simulink model "Controller29_05"  (R2019b)
settings: Solver=VariableStepAuto  StartTime=0.0  StopTime=10.0  RelTol=1e-3
undefined symbols (not defined in the file): maxsteer, x_p, y_p
settings Model: Creator=s161230  LastModifiedBy=s161230

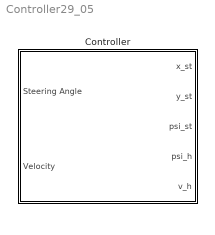
== system Controller29_05 ==
  Controller : Subsystem

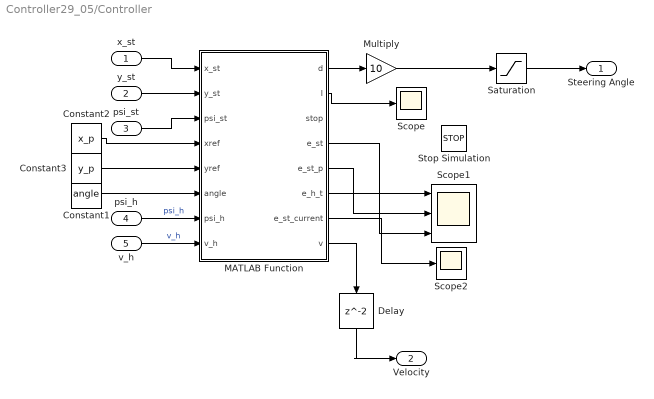
== system Controller29_05/Controller ==
  x_st : Inport  OutDataTypeStr=double
  y_st : Inport  Port=2  OutDataTypeStr=double
  psi_st : Inport  Port=3  OutDataTypeStr=double
  psi_h : Inport  Port=4  OutDataTypeStr=double
  v_h : Inport  Port=5  OutDataTypeStr=double
  Constant1 : Constant  Value=angle
  Constant2 : Constant  Value=x_p
  Constant3 : Constant  Value=y_p
  Delay : Delay  InitialCondition=-1.0
  MATLAB Function : MATLAB Function  TreatAsAtomicUnit=on
  Multiply : Gain  Gain=10
  Saturation : Saturate  UpperLimit=maxsteer  LowerLimit=-maxsteer  ZeroCross=off
  Scope : Scope
  Scope1 : Scope  NumInputPorts=3
  Scope2 : Scope
  Stop Simulation : Stop
  Steering Angle : Outport  OutDataTypeStr=double
  "Velocity " : Outport  Port=2
  wires:
  Constant1/1 -> MATLAB Function/6(angle)
  MATLAB Function/1(d) -> Multiply/1
  Constant2/1 -> MATLAB Function/4(xref)
  psi_st/1 -> MATLAB Function/3(psi_st)
  Constant3/1 -> MATLAB Function/5(yref)
  x_st/1 -> MATLAB Function/1(x_st)
  y_st/1 -> MATLAB Function/2(y_st)
  psi_h/1 -> MATLAB Function/7(psi_h)  "psi_h"
  v_h/1 -> MATLAB Function/8(v_h)  "v_h"
  Multiply/1 -> Saturation/1
  MATLAB Function/2(I) -> Scope/1
  MATLAB Function/4(e_st) -> Scope1/1
  MATLAB Function/5(e_st_p) -> Scope1/2
  MATLAB Function/6(e_h_t) -> Scope1/3
  Saturation/1 -> Steering Angle/1
  MATLAB Function/7(e_st_current) -> Scope2/1
  MATLAB Function/8(v) -> Delay/1
  Delay/1 -> "Velocity "/1

== matlab function Controller29_05/Controller/MATLAB Function ==
  data: d output; I output; stop output; x_st input; y_st input; psi_st input; xref input; yref input; angle input; psi_h input; v_h input; e_st output; e_st_p output; e_h_t output; e_st_current output; v output
function [d, I, stop, e_st, e_st_p, e_h_t, e_st_current, v]  = Error(x_st, y_st, psi_st, xref, yref, angle, psi_h,v_h)
    [~, I] = min(sqrt((xref-x_st).^2+(yref-y_st).^2));
    lookahead = 200;
    K1 = 80;%2
    K2 = 7.6;%13
    l_h = 0.22;
    l_st = 0.72;
    
    %1.0m
    lookahead = 77; %77
    K1 = 75;        %75
    K2 = 12;        %12
    
    %0.9m
    lookahead = 82;
    K1 = 76;
    K2 = 12;
    
    %0.8m
    lookahead = 86;
    K1 = 77;
    K2 = 12;
        
    %0.7m
    lookahead = 88;
    K1 = 79;
    K2 = 12;
    
    %0.6m
    lookahead = 95;
    K1 = 79;
    K2 = 12;
    
    %0.5m
    lookahead = 110;
    K1 = 79;
    K2 = 12;
    
    %0.4m
    lookahead = 150;
    K1 = 79;
    K2 = 12;
    
    %0.35m
%     lookahead = 210;
%     K1 = 86;
%     K2 = 12;
    
    %0.3m
%     lookahead = 220;
%     K1 = 90;
%     K2 = 12;
%     
    if I < length(angle) - 1
        stop = 0;
        
        if I < length(angle) - lookahead
            
             e_st_current = -sin(psi_st)*(x_st-xref(I))+cos(psi_st)*(y_st-yref(I));
             %define errors
             e_st = -sin(psi_st)*(x_st-xref(I+lookahead))+cos(psi_st)*(y_st-yref(I+lookahead));
             e_st = -sin(psi_st)*(-x_st+xref(I+lookahead))+cos(psi_st)*(-y_st+yref(I+lookahead));

             e_st_p = psi_st - angle(I+lookahead);
             
             %difference heading truck and heading trailer
             e_h_t = psi_h-psi_st;
             
             %desired value for e_h_t (input u)
             u = -atan((l_st/v_h)*(K1*e_st_p/cos(e_h_t)+e_st*v_h*sin(e_st_p)/e_st_p));
             
             %dynamics
             e_st_p_dot = v_h/l_st*sin(e_h_t);
             e_st_dot = v_h*cos(e_h_t)*sin(e_st_p);
             u_dot = -1*(1/(1+((l_st/v_h)*K1*e_st_p/cos(e_h_t)+e_st*v_h*sin(e_st_p)/e_st_p)^2))*(l_st/v_h)*(K1*e_st_p_dot/cos(e_h_t)+e_st_dot*v_h*sin(e_st_p)/e_st_p+e_st*v_h*e_st_p_dot*(cos(e_st_p)*e_st_p-sin(e_st_p))/(e_st_p^2));
    
             %difference between desired and actual
             z = (psi_h-psi_st)-u;
             
             %steering angle to achieve required path
             d = asin((l_h/v_h)*(-K2*z+u_dot+(v_h/l_st)*sin(psi_h-psi_st)));
             %trying something
%              d = atan((l_h/v_h)*(-K2*u+v_h/l_st*tan(e_h_t)*cos(e_h_t)));
             v = -1;
        else
            %define erros
             e_st_current = -sin(psi_st)*(x_st-xref(I))+cos(psi_st)*(y_st-yref(I));
             e_st = -sin(psi_st)*(x_st-xref(end))+cos(psi_st)*(y_st-yref(end));
             e_st = -sin(psi_st)*(-x_st+xref(end))+cos(psi_st)*(-y_st+yref(end));

             e_st_p = psi_st - angle(end);
             
             %difference heading truck and heading trailer
             e_h_t = psi_h-psi_st;
             
             %desired value for e_h_t (input u)
             u = -atan((l_st/v_h)*(K1*e_st_p/cos(e_h_t)+e_st*v_h*sin(e_st_p)/e_st_p));
             
             %dynamics
             e_st_p_dot = v_h/l_st*sin(e_h_t);
             e_st_dot = v_h*cos(e_h_t)*sin(e_st_p);
             u_dot = -1*(1/(1+((l_st/v_h)*K1*e_st_p/cos(e_h_t)+e_st*v_h*sin(e_st_p)/e_st_p)^2))*(l_st/v_h)*(K1*e_st_p_dot/cos(e_h_t)+e_st_dot*v_h*sin(e_st_p)/e_st_p+e_st*v_h*e_st_p_dot*(cos(e_st_p)*e_st_p-sin(e_st_p))/(e_st_p^2));
             
             %difference between desired and actual
             z = (psi_h-psi_st)-u;
             
             %steering angle to achieve required path
             d = asin((l_h/v_h)*(-K2*z+u_dot+(v_h/l_st)*sin(psi_h-psi_st)));
             v = -0.2;
        end
    else
        e_st_current = 0;
        e_st = 0;
        e_st_p = 0;
        e_h_t = 0;
        d = 0;
        stop = 1;
        v = 0;
    end
end
